simulink model "simple_model"  (R2019a)
settings: Solver=VariableStepAuto  StartTime=0.0  StopTime=10.0  RelTol=1e-3
settings Model: Creator=rosha  LastModifiedBy=rosha

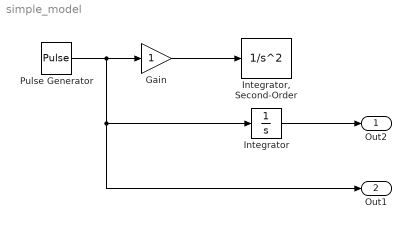
== system simple_model ==
  Gain : Gain
  Integrator : Integrator
  "Integrator, Second-Order" : SecondOrderIntegrator
  Pulse Generator : DiscretePulseGenerator  PulseType=Time based  Amplitude=5  Period=10  PulseWidth=20  PhaseDelay=2
  Out2 : Outport
  Out1 : Outport  Port=2
  wires:
  Gain/1 -> "Integrator, Second-Order"/1
  Pulse Generator/1 -> Out1/1, Integrator/1, Gain/1
  Integrator/1 -> Out2/1
